simulink model "initial_conditions"  (R2019b)
settings: Solver=FixedStepAuto  StartTime=0.0  StopTime=100  FixedStep=0.001  RelTol=1e-3
settings Model: Creator=davis  LastModifiedBy=davis

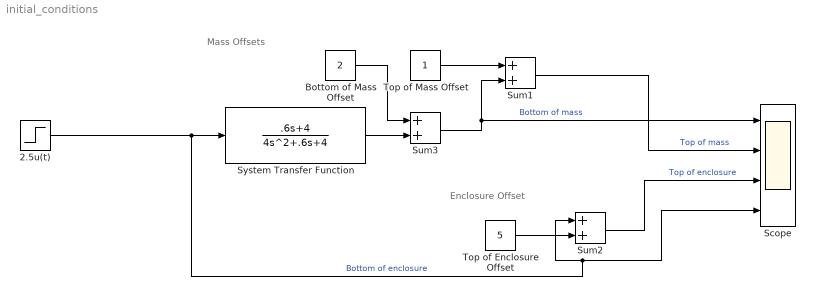
== system initial_conditions ==
  note: Mass Offsets
  note: Enclosure Offset
  2.5u(t) : Step  Time=0  After=2.5  SampleTime=0
  Bottom of Mass Offset : Constant  Value=2
  Scope : Scope  NumInputPorts=4
  Sum1 : Sum
  Sum2 : Sum
  Sum3 : Sum
  System Transfer Function : TransferFcn  Numerator=[.6 4]  Denominator=[4 .6 4]
  Top of Enclosure Offset : Constant  Value=5
  Top of Mass Offset : Constant
  wires:
  Top of Enclosure Offset/1 -> Sum2/2
  2.5u(t)/1 -> Scope/4, Sum2/1, System Transfer Function/1  "Bottom of enclosure"
  Bottom of Mass Offset/1 -> Sum3/1
  System Transfer Function/1 -> Sum3/2
  Sum3/1 -> Scope/1, Sum1/2  "Bottom of mass"
  Sum1/1 -> Scope/2  "Top of mass"
  Sum2/1 -> Scope/3  "Top of enclosure"
  Top of Mass Offset/1 -> Sum1/1
